simulink model "ApogeeCompletedSimulinkModel"  (R2024b)
settings: Solver=VariableStepAuto  StartTime=0.0  StopTime=10.0  RelTol=1e-3
libraries: simulink x2
settings Model: Creator=Vaiebhav  LastModifiedBy=GIRISHRAO JADHAVRAO

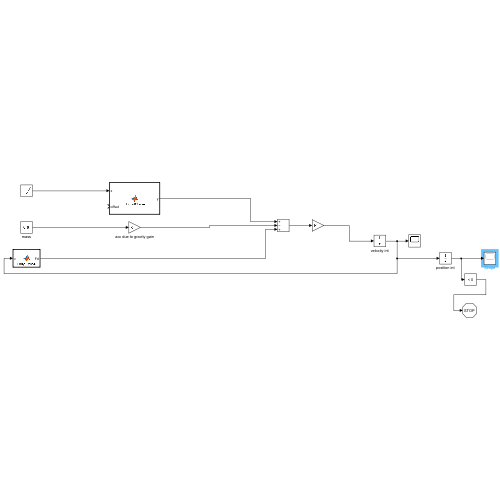
[thumbnail: Simulink's stored preview of the top-level diagram]
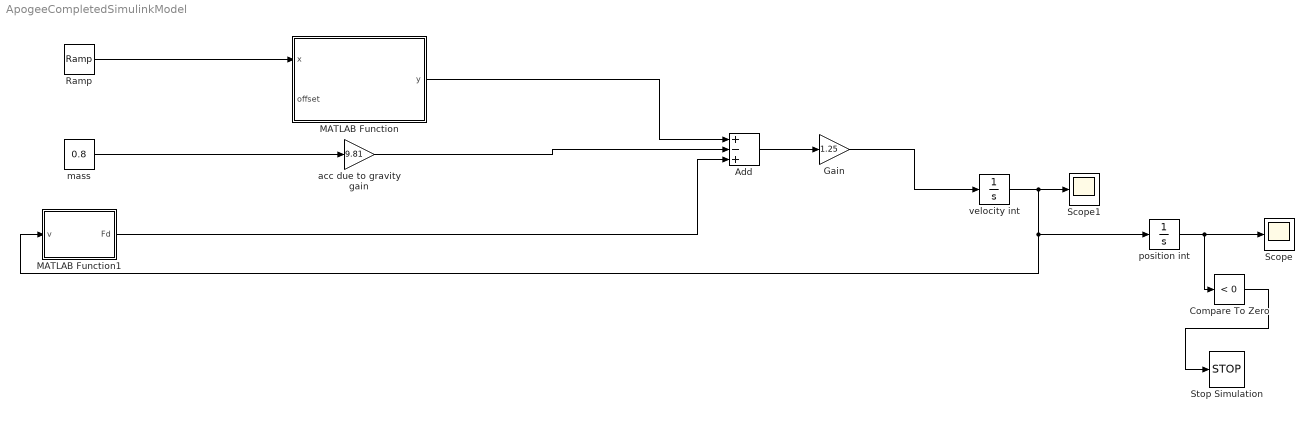
== system ApogeeCompletedSimulinkModel ==
  Add : Sum  Inputs=+-+
  Compare To Zero : simulink/Logic and Bit Operations/Compare To Zero  relop=<  OutDataTypeStr=boolean
  Gain : Gain  Gain=1.25
  MATLAB Function : MATLAB Function  TreatAsAtomicUnit=on
  MATLAB Function1 : MATLAB Function  TreatAsAtomicUnit=on
  Ramp : simulink/Sources/Ramp  slope=1  start=0  InitialOutput=0
  Scope : Scope
  Scope1 : Scope
  Stop Simulation : Stop
  acc due to gravity gain : Gain  Gain=9.81
  mass : Constant  Value=0.8
  position int : Integrator  InitialCondition=0.1
  velocity int : Integrator
  wires:
  mass/1 -> acc due to gravity gain/1
  acc due to gravity gain/1 -> Add/2
  MATLAB Function/1(y) -> Add/1
  Add/1 -> Gain/1
  Ramp/1 -> MATLAB Function/1(x)
  Gain/1 -> velocity int/1
  velocity int/1 -> Scope1/1, position int/1, MATLAB Function1/1(v)
  position int/1 -> Compare To Zero/1, Scope/1
  MATLAB Function1/1(Fd) -> Add/3
  Compare To Zero/1 -> Stop Simulation/1

== matlab function ApogeeCompletedSimulinkModel/MATLAB Function ==
  data: x input; y output; offset input
function y = ThrustCurve(x, offset)
    if x >= offset && x <= 0.25 + offset
        y = 120*(x-offset);
    elseif x >= 0.25 + offset && x <= 1 + offset
        %y = 10.0503 + 0.0847658/((x-offset)^3.94032);
        %y = -20213 + 20226.1/(x-offset)^0.0000294692;
        y = 9.9672 + 1311.23*exp(-14.5652*(x-offset));
    elseif x >= 1 + offset && x <= 2.8 + offset
        y = 10;
    else
        y = 0;
    end
end

== matlab function ApogeeCompletedSimulinkModel/MATLAB Function1 ==
  data: v input; Fd output
function Fd = DragForce(v)
if v>=0
    Cd = 0.5; % Example drag coefficient
    A = 0.01; % Example cross-sectional area in m²
    rho = 1.225; % Air density in kg/m³
    Fd = -0.5 * Cd * A * rho * v * v;
    
else
        
          Cd = 1.5;
          A = 0.5;
          rho = 1.225;
           Fd = 0.5 * Cd * A * rho * v * v;
        
end
end
